simulink model "COGAG"  (Simulink 8.3)
settings: Solver=ode45  StartTime=0.0  StopTime=100.0  FixedStep=0.1  RelTol=1e-3
libraries: simulink_need_slupdate x2
(part 1 of 3)
settings Model: Creator=Administrator  LastModifiedBy=Administrator
settings DataIOCC: SignalLoggingSaveFormat=Dataset  InspectSignalLogs=on
settings DebuggingCC: UnderspecifiedInitializationDetection=Simplified  StateNameClashWarn=none
settings GRTTargetCC: CombineOutputUpdateFcns=on  GRTInterface=off

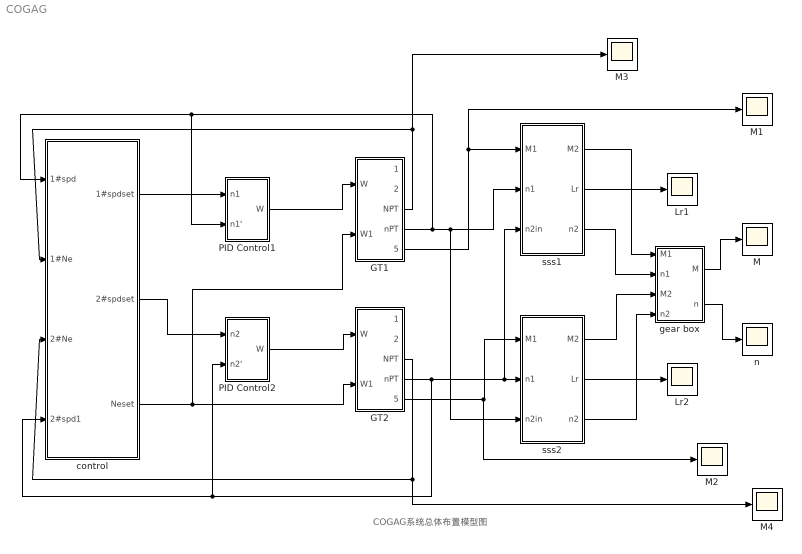
== system COGAG ==
  note: COGAG系统总体布置模型图
  GT1 : Subsystem
  GT2 : Subsystem
  Lr1 : Scope
      settings: YMin=0  YMax=15  SaveName=ScopeData2
  Lr2 : Scope
      settings: SaveName=ScopeData5
  M{,1..4} (5 alike) : Scope
      M settings: SaveName=ScopeData6
      M1 settings: SaveName=ScopeData11
      M2 settings: SaveName=ScopeData12
      M3 settings: SaveName=ScopeData13
      M4 settings: SaveName=ScopeData19
  PID Control1 : Subsystem
  PID Control2 : Subsystem
  control : Subsystem
  gear box : Subsystem
  n : Scope
      settings: SaveName=ScopeData8
  sss1 : Subsystem
  sss2 : Subsystem
  wires:
  GT1/4(nPT) -> sss1/2(n1), sss2/3(n2in), PID Control1/2(n1'), control/1(1#spd)
  GT2/4(nPT) -> control/4(2#spd1), PID Control2/2(n2'), sss2/2(n1), sss1/3(n2in)
  PID Control1/1(W) -> GT1/1(W)
  PID Control2/1(W) -> GT2/1(W)
  control/1(1#spdset) -> PID Control1/1(n1)
  control/2(2#spdset) -> PID Control2/1(n2)
  control/3(Neset) -> GT2/2(W1), GT1/2(W1)
  GT1/3(NPT) -> M3/1, control/2(1#Ne)
  GT2/3(NPT) -> M4/1, control/3(2#Ne)
  GT1/5(MPT) -> M1/1, sss1/1(M1)
  GT2/5(MPT) -> M2/1, sss2/1(M1)
  sss1/2(Lr) -> Lr1/1
  sss2/2(Lr) -> Lr2/1
  gear box/1(M) -> M/1
  gear box/2(n) -> n/1
  sss2/3(n2) -> gear box/4(n2)
  sss1/1(M2) -> gear box/1(M1)
  sss1/3(n2) -> gear box/2(n1)
  sss2/1(M2) -> gear box/3(M2)

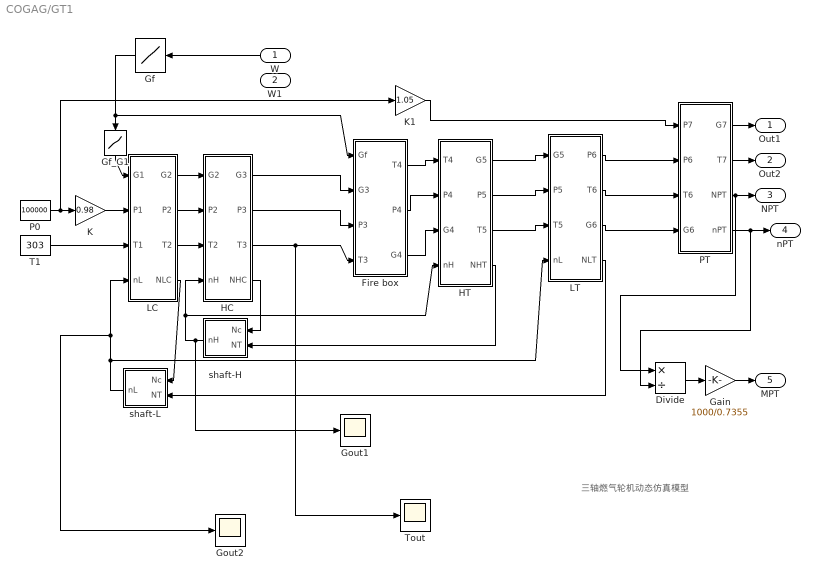
== system COGAG/GT1 ==
  note: 三轴燃气轮机动态仿真模型
  W : Inport
  W1 : Inport  Port=2
  Divide : Product  Inputs=*/
  Fire box : Subsystem
  Gain : Gain  Gain=1000/0.7355
  Gf : Lookup  InputValues=[0,0.03,0.07,0.09,0.11,0.13,0.17,0.2,0.23,0.26,0.28,0.3,0.32,0.34,0.35,0.38,0.4,0.42,0.44,0.47,0.49,0.5,0.52,0.54,0.55,0.59,0.61,0.64,0.66,0.68,0.7,0.72,0.74,0.77,0.81,0.83,0.85,0.88,0.93,0.95,0.97,1]  Table=[0.172,0.236,0.331,0.331,0.366,0.411,0.488,0.536,0.582,0.605,0.644,0.682,0.698,0.728,0.727,0.783,0.783,0.813,0.857,0.886,0.935,0.949,0.95,0.975,0.999,1.022,1.069,1.149,1.153,1.184,1.206,1.233,1.256,1.271,1.325,1.383,1.383,1.439,1.481,1.504,1.52,1.574]
  Gf_G1 : Lookup  InputValues=[0.172,0.236,0.331,0.366,0.411,0.488,0.536,0.582,0.605,0.644,0.682,0.698,0.727,0.728,0.783,0.813,0.857,0.886,0.935,0.949,0.95,0.975,0.999,1.022,1.069,1.149,1.153,1.184,1.206,1.233,1.256,1.271,1.325,1.383,1.439,1.481,1.504,1.52,1.574]  Table="[20.01, 25.93, 38.77,  43.65, 45.94, 51.85, 54.70, 56.85, 59.03, 61.91, 60.44, 61.58, 62.93, 63.04, 65.71,   67.00, 69.52, 70.63, 73.19, 73.46, 73.44, 73.83, 75.62, 76.39, 78.27, 81.17, 81.50, 82.44, 83.44, 84.31, 85.30, 86.17, 87.93, 89.72, 91.51, 93.65, 94.63, 94.92, 97.64]"
  Gout1 : Scope
      settings: TimeRange=10
  Gout2 : Scope
      settings: TimeRange=10  SaveName=ScopeData3
  HC : Subsystem
  HT : Subsystem
  K : Gain  Gain=0.98
  K1 : Gain  Gain=1.05
  LC : Subsystem
  LT : Subsystem
  P0 : Constant  Value=100000
  PT : Subsystem
  T1 : Constant  Value=303
  Tout : Scope
      settings: TimeRange=200  YMin=740  YMax=790
  shaft-H : Subsystem  mask(rotor module){J=30}
      mask prompts: J "J moment of inertia(Nm)"
      mask help: (pi^2*J*n/900)*(dn/dt)=NT-Nc
  shaft-L : Subsystem  mask(rotor module){J=15}
      mask prompts: J "J moment of inertia(Nm)"
      mask help: (pi^2*J*n/900)*(dn/dt)=NT-Nc
  Out1 : Outport
  Out2 : Outport  Port=2
  NPT : Outport  Port=3
  nPT : Outport  Port=4
  MPT : Outport  Port=5
  wires:
  T1/1 -> LC/3(T1)
  K/1 -> LC/2(P1)
  LC/1(G2) -> HC/1(G2)
  LC/2(P2) -> HC/2(P2)
  LC/3(T2) -> HC/3(T2)
  HC/1(G3) -> Fire box/2(G3)
  HC/2(P3) -> Fire box/3(P3)
  HC/3(T3) -> Fire box/4(T3), Tout/1
  HC/4(NHC) -> shaft-H/1(Nc)
  HT/4(NHT) -> shaft-H/2(NT)
  shaft-H/1(nH) -> HT/4(nH), HC/4(nH), Gout1/1
  LC/4(NLC) -> shaft-L/1(Nc)
  LT/4(NLT) -> shaft-L/2(NT)
  Gf/1 -> Gf_G1/1, Fire box/1(Gf)
  Gf_G1/1 -> LC/1(G1)
  Fire box/3(G4) -> HT/3(G4)
  Fire box/2(P4) -> HT/2(P4)
  HT/3(T5) -> LT/3(T5)
  HT/2(P5) -> LT/2(P5)
  HT/1(G5) -> LT/1(G5)
  LT/3(G6) -> PT/4(G6)
  LT/2(T6) -> PT/3(T6)
  shaft-L/1(nL) -> LT/4(nL), LC/4(nL), Gout2/1
  LT/1(P6) -> PT/2(P6)
  P0/1 -> K/1, K1/1
  Fire box/1(T4) -> HT/1(T4)
  K1/1 -> PT/1(P7)
  W/1 -> Gf/1
  PT/1(G7) -> Out1/1
  PT/2(T7) -> Out2/1
  PT/3(NPT) -> NPT/1, Divide/1
  PT/4(nPT) -> nPT/1, Divide/2
  Gain/1 -> MPT/1
  Divide/1 -> Gain/1

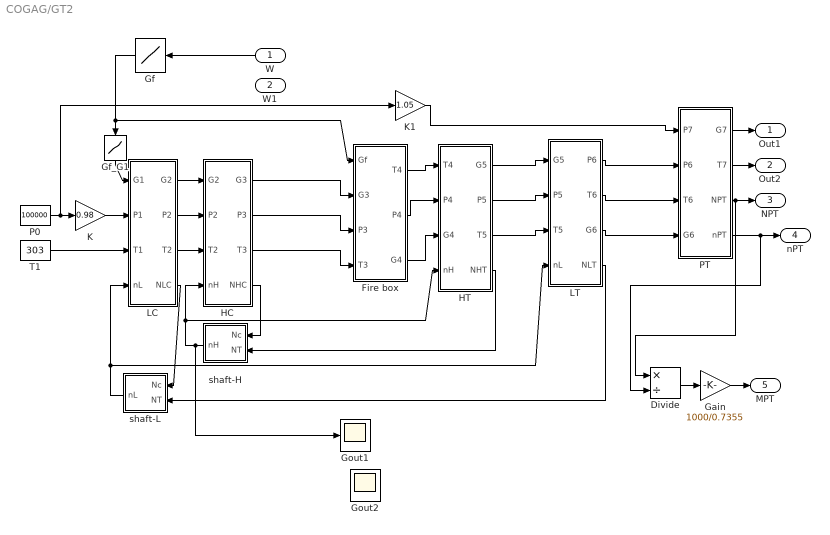
== system COGAG/GT2 ==
  W : Inport
  W1 : Inport  Port=2
  Divide : Product  Inputs=*/
  Fire box : Subsystem
  Gain : Gain  Gain=1000/0.7355
  Gf : Lookup  InputValues=[0,0.03,0.07,0.09,0.11,0.13,0.17,0.2,0.23,0.26,0.28,0.3,0.32,0.34,0.35,0.38,0.4,0.42,0.44,0.47,0.49,0.5,0.52,0.54,0.55,0.59,0.61,0.64,0.66,0.68,0.7,0.72,0.74,0.77,0.81,0.83,0.85,0.88,0.93,0.95,0.97,1]  Table=[0.172,0.236,0.331,0.331,0.366,0.411,0.488,0.536,0.582,0.605,0.644,0.682,0.698,0.728,0.727,0.783,0.783,0.813,0.857,0.886,0.935,0.949,0.95,0.975,0.999,1.022,1.069,1.149,1.153,1.184,1.206,1.233,1.256,1.271,1.325,1.383,1.383,1.439,1.481,1.504,1.52,1.574]
  Gf_G1 : Lookup  InputValues=[0.172,0.236,0.331,0.366,0.411,0.488,0.536,0.582,0.605,0.644,0.682,0.698,0.727,0.728,0.783,0.813,0.857,0.886,0.935,0.949,0.95,0.975,0.999,1.022,1.069,1.149,1.153,1.184,1.206,1.233,1.256,1.271,1.325,1.383,1.439,1.481,1.504,1.52,1.574]  Table="[20.01, 25.93, 38.77,  43.65, 45.94, 51.85, 54.70, 56.85, 59.03, 61.91, 60.44, 61.58, 62.93, 63.04, 65.71,   67.00, 69.52, 70.63, 73.19, 73.46, 73.44, 73.83, 75.62, 76.39, 78.27, 81.17, 81.50, 82.44, 83.44, 84.31, 85.30, 86.17, 87.93, 89.72, 91.51, 93.65, 94.63, 94.92, 97.64]"
  Gout1 : Scope
      settings: TimeRange=10
  Gout2 : Scope
      settings: TimeRange=10  SaveName=ScopeData26
  HC : Subsystem
  HT : Subsystem
  K : Gain  Gain=0.98
  K1 : Gain  Gain=1.05
  LC : Subsystem
  LT : Subsystem
  P0 : Constant  Value=100000
  PT : Subsystem
  T1 : Constant  Value=303
  shaft-H : Subsystem  mask(rotor module){J=30}
      mask prompts: J "J moment of inertia(Nm)"
      mask help: (pi^2*J*n/900)*(dn/dt)=NT-Nc
  shaft-L : Subsystem  mask(rotor module){J=15}
      mask prompts: J "J moment of inertia(Nm)"
      mask help: (pi^2*J*n/900)*(dn/dt)=NT-Nc
  Out1 : Outport
  Out2 : Outport  Port=2
  NPT : Outport  Port=3
  nPT : Outport  Port=4
  MPT : Outport  Port=5
  wires:
  T1/1 -> LC/3(T1)
  K/1 -> LC/2(P1)
  LC/1(G2) -> HC/1(G2)
  LC/2(P2) -> HC/2(P2)
  LC/3(T2) -> HC/3(T2)
  HC/1(G3) -> Fire box/2(G3)
  HC/2(P3) -> Fire box/3(P3)
  HC/3(T3) -> Fire box/4(T3)
  HC/4(NHC) -> shaft-H/1(Nc)
  HT/4(NHT) -> shaft-H/2(NT)
  shaft-H/1(nH) -> HT/4(nH), HC/4(nH), Gout1/1
  LC/4(NLC) -> shaft-L/1(Nc)
  LT/4(NLT) -> shaft-L/2(NT)
  Gf/1 -> Gf_G1/1, Fire box/1(Gf)
  Gf_G1/1 -> LC/1(G1)
  Fire box/3(G4) -> HT/3(G4)
  Fire box/2(P4) -> HT/2(P4)
  HT/3(T5) -> LT/3(T5)
  HT/2(P5) -> LT/2(P5)
  HT/1(G5) -> LT/1(G5)
  LT/3(G6) -> PT/4(G6)
  LT/2(T6) -> PT/3(T6)
  shaft-L/1(nL) -> LT/4(nL), LC/4(nL)
  LT/1(P6) -> PT/2(P6)
  P0/1 -> K/1, K1/1
  Fire box/1(T4) -> HT/1(T4)
  K1/1 -> PT/1(P7)
  W/1 -> Gf/1
  PT/1(G7) -> Out1/1
  PT/2(T7) -> Out2/1
  PT/3(NPT) -> NPT/1, Divide/1
  PT/4(nPT) -> nPT/1, Divide/2
  Gain/1 -> MPT/1
  Divide/1 -> Gain/1

== system COGAG/PID Control1 ==
  note: 模糊自整定PID控制器
  n1 : Inport
  n1' : Inport  Port=2
  Add : Sum  Inputs=+-
  PID Controller : simulink_need_slupdate/PID Controller  P=0.006  I=10  D=0
  Transfer Fcn : TransferFcn  Denominator=[0.6 1]
  W : Outport
  wires:
  Add/1 -> PID Controller/1
  Transfer Fcn/1 -> W/1
  n1/1 -> Add/1
  n1'/1 -> Add/2
  PID Controller/1 -> Transfer Fcn/1

== system COGAG/PID Control2 ==
  n2 : Inport
  n2' : Inport  Port=2
  Add : Sum  Inputs=+-
  PID Controller : simulink_need_slupdate/PID Controller  P=0.006  I=10  D=0
  Transfer Fcn : TransferFcn  Denominator=[0.6 1]
  W : Outport
  wires:
  Add/1 -> PID Controller/1
  PID Controller/1 -> Transfer Fcn/1
  Transfer Fcn/1 -> W/1
  n2/1 -> Add/1
  n2'/1 -> Add/2

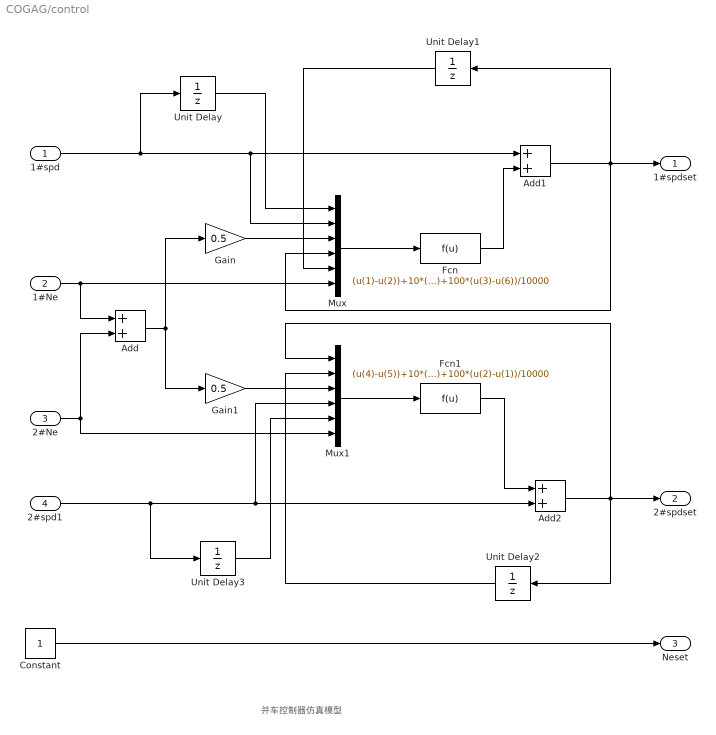
== system COGAG/control ==
  note: 并车控制器仿真模型
  1#spd : Inport
  1#Ne : Inport  Port=2
  2#Ne : Inport  Port=3
  2#spd1 : Inport  Port=4
  Add : Sum
  Add1 : Sum
  Add2 : Sum
  Constant : Constant
  Fcn : Fcn  Expr=(u(1)-u(2))+10*((u(1)-u(2))+u(4)-u(5))+100*(u(3)-u(6))/10000
  Fcn1 : Fcn  Expr=(u(4)-u(5))+10*((u(4)-u(5))+u(4)-u(5))+100*(u(2)-u(1))/10000
  Gain : Gain  Gain=0.5
  Gain1 : Gain  Gain=0.5
  Mux : Mux  Inputs=6
  Mux1 : Mux  Inputs=6
  Unit Delay{,1..3} (4 alike) : UnitDelay  SampleTime=0.02
  1#spdset : Outport
  2#spdset : Outport  Port=2
  Neset : Outport  Port=3
  wires:
  1#Ne/1 -> Add/1, Mux/6
  2#Ne/1 -> Add/2, Mux1/6
  Add/1 -> Gain/1, Gain1/1
  Gain/1 -> Mux/3
  Fcn/1 -> Add1/2
  1#spd/1 -> Unit Delay/1, Add1/1, Mux/2
  Unit Delay/1 -> Mux/1
  Add1/1 -> Mux/4, Unit Delay1/1, 1#spdset/1
  Gain1/1 -> Mux1/3
  Add2/1 -> Unit Delay2/1, 2#spdset/1, Mux1/1
  2#spd1/1 -> Unit Delay3/1, Add2/2, Mux1/4
  Fcn1/1 -> Add2/1
  Unit Delay2/1 -> Mux1/2
  Unit Delay3/1 -> Mux1/5
  Constant/1 -> Neset/1
  Unit Delay1/1 -> Mux/5
  Mux/1 -> Fcn/1
  Mux1/1 -> Fcn1/1

== system COGAG/gear box ==
  note: 并车齿轮箱模型
  M1 : Inport
  n1 : Inport  Port=2
  M2 : Inport  Port=3
  n2 : Inport  Port=4
  Add : Sum
  Fcn : Fcn  Expr=1/u
  Gain : Gain  Gain=1/3.5
  Product : Product
  Product1 : Product
  Product2 : Product
  M : Outport
  n : Outport  Port=2
  wires:
  M1/1 -> Product/1
  n1/1 -> Gain/1, Product/2
  Product/1 -> Add/1
  M2/1 -> Product1/1
  n2/1 -> Product1/2
  Product1/1 -> Add/2
  Gain/1 -> n/1, Fcn/1
  Add/1 -> Product2/1
  Fcn/1 -> Product2/2
  Product2/1 -> M/1

== system COGAG/sss1 ==
  note: sss离合器模块
  M1 : Inport
  n1 : Inport  Port=2
  n2in : Inport  Port=3
  Add : Sum  Inputs=+-
  Fcn : Fcn  Expr=u*pi/30
  Subsystem : Subsystem
  Subsystem1 : Subsystem
  Subsystem2 : Subsystem
  Subsystem3 : Subsystem
  Switch : Switch
  M2 : Outport
  Lr : Outport  Port=2
  n2 : Outport  Port=3
  wires:
  n1/1 -> Subsystem3/2(n1), Switch/1
  Fcn/1 -> Add/2
  Switch/1 -> n2/1
  M1/1 -> Subsystem3/1(M1)
  Subsystem/1(J1) -> Subsystem3/3(J1)
  Subsystem/2(Jz) -> Subsystem1/2(Jz)
  Subsystem3/1(Mfzf) -> Subsystem1/1(Mfzf)
  Subsystem3/3(C1) -> Subsystem1/3(C1)
  Subsystem1/1(Mr) -> Subsystem2/1(Mr)
  Subsystem1/3(C2) -> Subsystem2/3(C2)
  Subsystem1/2(Lr) -> Switch/2, Lr/1
  Subsystem3/2(wf) -> Add/1
  Subsystem/3(J2) -> Subsystem2/2(J2)
  Subsystem2/1(M2) -> M2/1
  Subsystem/4(f) -> Subsystem1/4(f)
  n2in/1 -> Subsystem2/4(n2in)
  Add/1 -> Subsystem1/5(Wz)
  Subsystem2/2(n2) -> Fcn/1, Switch/3

== system COGAG/sss2 ==
  note: sss离合器模块
  M1 : Inport
  n1 : Inport  Port=2
  n2in : Inport  Port=3
  Add : Sum  Inputs=+-
  Fcn : Fcn  Expr=u*pi/30
  Subsystem : Subsystem
  Subsystem1 : Subsystem
  Subsystem2 : Subsystem
  Subsystem3 : Subsystem
  Switch : Switch
  M2 : Outport
  Lr : Outport  Port=2
  n2 : Outport  Port=3
  wires:
  n1/1 -> Subsystem3/2(n1), Switch/1
  Fcn/1 -> Add/2
  Switch/1 -> n2/1
  M1/1 -> Subsystem3/1(M1)
  Subsystem/1(J1) -> Subsystem3/3(J1)
  Subsystem/2(Jz) -> Subsystem1/2(Jz)
  Subsystem3/1(Mfzf) -> Subsystem1/1(Mfzf)
  Subsystem3/3(C1) -> Subsystem1/3(C1)
  Subsystem1/1(Mr) -> Subsystem2/1(Mr)
  Subsystem1/3(C2) -> Subsystem2/3(C2)
  Subsystem1/2(Lr) -> Switch/2, Lr/1
  Subsystem3/2(wf) -> Add/1
  Subsystem/3(J2) -> Subsystem2/2(J2)
  Subsystem2/1(M2) -> M2/1
  Subsystem/4(f) -> Subsystem1/4(f)
  n2in/1 -> Subsystem2/4(n2in)
  Add/1 -> Subsystem1/5(Wz)
  Subsystem2/2(n2) -> Fcn/1, Switch/3

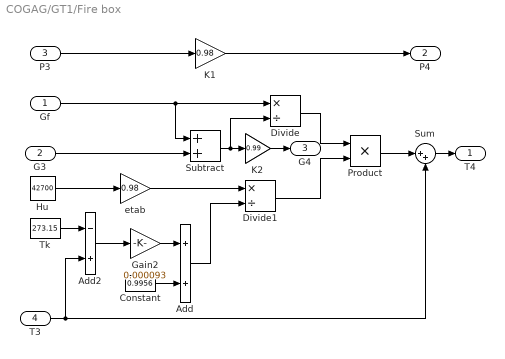
== system COGAG/GT1/Fire box ==
  Gf : Inport
  G3 : Inport  Port=2
  P3 : Inport  Port=3
  T3 : Inport  Port=4
  Add : Sum
  Add2 : Sum  Inputs=-+
  Constant : Constant  Value=0.9956
  Divide : Product  Inputs=*/
  Divide1 : Product  Inputs=*/
  Gain2 : Gain  Gain=0.000093
  Hu : Constant  Value=42700
  K1 : Gain  Gain=0.98
  K2 : Gain  Gain=0.99
  Product : Product  RndMeth=Zero
  Subtract : Sum
  Sum : Sum  Inputs=|++
  Tk : Constant  Value=273.15
  etab : Gain  Gain=0.98
  T4 : Outport
  P4 : Outport  Port=2
  G4 : Outport  Port=3
  wires:
  Gf/1 -> Divide/1, Subtract/1
  Divide/1 -> Product/1
  G3/1 -> Subtract/2
  Subtract/1 -> Divide/2, K2/1
  Hu/1 -> etab/1
  etab/1 -> Divide1/1
  Divide1/1 -> Product/2
  Product/1 -> Sum/1
  Sum/1 -> T4/1
  T3/1 -> Add2/2, Sum/2
  P3/1 -> K1/1
  K1/1 -> P4/1
  Constant/1 -> Add/2
  Gain2/1 -> Add/1
  Tk/1 -> Add2/1
  Add2/1 -> Gain2/1
  Add/1 -> Divide1/2
  K2/1 -> G4/1

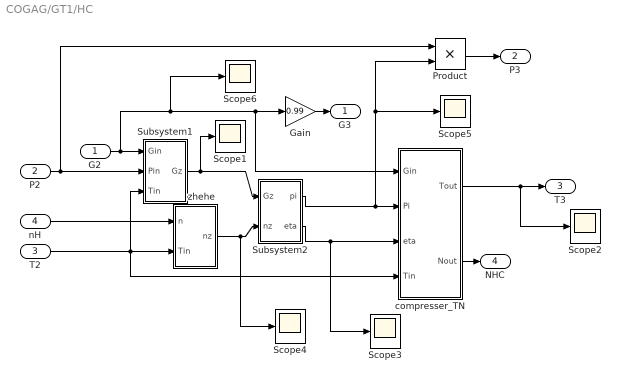
== system COGAG/GT1/HC ==
  G2 : Inport
  P2 : Inport  Port=2
  T2 : Inport  Port=3
  nH : Inport  Port=4
  Gain : Gain  Gain=0.99
  Product : Product  RndMeth=Zero
  Scope{1..6} (6 alike) : Scope
      Scope1 settings: YMin=2829.54  YMax=3127.38  SaveName=ScopeData16
      Scope2 settings: YMin=2829.54  YMax=3127.38  SaveName=ScopeData29
      Scope3 settings: YMin=2829.54  YMax=3127.38  SaveName=ScopeData24
      Scope4 settings: YMin=2829.54  YMax=3127.38  SaveName=ScopeData31
      Scope5 settings: YMin=2829.54  YMax=3127.38  SaveName=ScopeData10
      Scope6 settings: YMin=2829.54  YMax=3127.38  SaveName=ScopeData15
  Subsystem1 : Subsystem
  Subsystem2 : Subsystem
  compresser_TN : Subsystem  mask(Compressor_Tout Nout module){}
  zhehe : Subsystem
  G3 : Outport
  P3 : Outport  Port=2
  T3 : Outport  Port=3
  NHC : Outport  Port=4
  wires:
  zhehe/1(nz) -> Scope4/1, Subsystem2/2(nz)
  Subsystem2/1(pi) -> compresser_TN/2(Pi), Product/2, Scope5/1
  Subsystem2/2(eta) -> compresser_TN/3(eta), Scope3/1
  T2/1 -> zhehe/2(Tin), compresser_TN/4(Tin), Subsystem1/3(Tin)
  nH/1 -> zhehe/1(n)
  Gain/1 -> G3/1
  compresser_TN/1(Tout) -> T3/1, Scope2/1
  compresser_TN/2(Nout) -> NHC/1
  Subsystem1/1(Gz) -> Scope1/1, Subsystem2/1(Gz)
  G2/1 -> Subsystem1/1(Gin), Gain/1, compresser_TN/1(Gin), Scope6/1
  P2/1 -> Subsystem1/2(Pin), Product/1
  Product/1 -> P3/1

== system COGAG/GT1/HT ==
  T4 : Inport
  P4 : Inport  Port=2
  G4 : Inport  Port=3
  nH : Inport  Port=4
  Divide : Product  Inputs=*/
  Scope3 : Scope
      settings: TimeRange=100  YMin=5000  YMax=25000  SaveName=ScopeData34
  n2-etaH : Lookup  InputValues=[6000 6300 6500 6800 7000 7150 7300 7500 7800]  Table=[0.81 0.83 0.85 0.87 0.88 0.87 0.86 0.855 0.85]
  n2-p1 : Lookup  InputValues=[6000 6503 6995 7498 8002 8505 8997 9500]  Table=[139400 150700 186000 246700 332500 443400 575800 736100]
  n2-p5 : Lookup  InputValues=[5832,7212,7282,7644,7752,7853,8033,8092 8211 8392 8430 8452 8670 8767 8960 8999 9073]  Table=[154000,269000,296000,361000,391000,419000,476000,494000 534000 596000 609000 616000 684000 719000 806000 814000 831000]
  pi : Scope
      settings: TimeRange=100  YMin=2829.54  YMax=3127.38  SaveName=ScopeData17
  pi1 : Scope
      settings: TimeRange=100  YMin=2829.54  YMax=3127.38  SaveName=ScopeData7
  pi2 : Scope
      settings: TimeRange=100  YMin=2829.54  YMax=3127.38  SaveName=ScopeData35
  turbine_TN : Subsystem  mask(Turbine_Tout Nout module){}
  G5 : Outport
  P5 : Outport  Port=2
  T5 : Outport  Port=3
  NHT : Outport  Port=4
  wires:
  n2-etaH/1 -> turbine_TN/2(eta)
  P4/1 -> Divide/1
  nH/1 -> pi2/1, n2-etaH/1, n2-p5/1
  turbine_TN/1(Tout) -> T5/1, pi1/1
  T4/1 -> turbine_TN/3(Tin)
  turbine_TN/2(Nout) -> NHT/1
  G4/1 -> turbine_TN/4(Gin), G5/1
  Divide/1 -> turbine_TN/1(Pi), pi/1
  n2-p5/1 -> Divide/2, P5/1, Scope3/1

== system COGAG/GT1/LC ==
  G1 : Inport
  P1 : Inport  Port=2
  T1 : Inport  Port=3
  nL : Inport  Port=4
  Gain : Gain  Gain=0.99
  Product : Product  RndMeth=Zero
  Scope{1..4} (4 alike) : Scope
      Scope1 settings: YMin=2829.54  YMax=3127.38  SaveName=ScopeData14
      Scope2 settings: YMin=2829.54  YMax=3127.38  SaveName=ScopeData9
      Scope3 settings: YMin=2829.54  YMax=3127.38  SaveName=ScopeData30
      Scope4 settings: TimeRange=80  YMin=5000  YMax=30000  SaveName=ScopeData32
  Subsystem1 : Subsystem
  Subsystem3 : Subsystem
  compresser_TN : Subsystem  mask(Compressor_Tout Nout module){}
  zhehe : Subsystem
  G2 : Outport
  P2 : Outport  Port=2
  T2 : Outport  Port=3
  NLC : Outport  Port=4
  wires:
  zhehe/1(nz) -> Scope1/1, Subsystem3/2(nz)
  Subsystem3/1(pi) -> compresser_TN/2(Pi), Product/2, Scope2/1
  Subsystem3/2(eta) -> compresser_TN/3(eta)
  T1/1 -> zhehe/2(Tin), compresser_TN/4(Tin), Subsystem1/3(Tin)
  nL/1 -> zhehe/1(n)
  Gain/1 -> G2/1
  compresser_TN/1(Tout) -> T2/1, Scope4/1
  compresser_TN/2(Nout) -> NLC/1
  Subsystem1/1(Gz) -> Scope3/1, Subsystem3/1(Gz)
  G1/1 -> Subsystem1/1(Gin), Gain/1, compresser_TN/1(Gin)
  P1/1 -> Subsystem1/2(Pin), Product/1
  Product/1 -> P2/1

== system COGAG/GT1/LT ==
  G5 : Inport
  P5 : Inport  Port=2
  T5 : Inport  Port=3
  nL : Inport  Port=4
  Divide : Product  Inputs=*/
  Scope1 : Scope
      settings: TimeRange=100  YMin=5000  YMax=25000  SaveName=ScopeData28
  Scope2 : Scope
      settings: TimeRange=100  YMin=5000  YMax=25000  SaveName=ScopeData4
  Scope3 : Scope
      settings: TimeRange=100  YMin=5000  YMax=25000  SaveName=ScopeData20
  n1-p1 : Lookup  InputValues="[2849,4651,4850,5410,5586,5742,6024,6092,6102,6211,6385,6425 6435 6609 6698  6732 7015  7080 7185 ]"  Table="[101000,131000,141000,161000,171000,181000,201000,201000,211000,221000,241000,251000 251000 281000 291000  301000 321000  331000 341000]"
  n1-p6 : Lookup  InputValues=[2849,4651,4850,5410,5586,5742,6024,6092,6102,6211,6385,6425,6435,6609,6698,6732,7015,7080,7185]  Table=[113000,150000,157000,180000,190000,201000,221000,229000,229500,242000,267000,272000,277000,306000,321000,322000,354000,360000,371000]
  n2-etaH : Lookup  InputValues=[4300 5000 5500 6000 6500 7000 7500 8000 9000 9500]  Table=[0.82 0.83 0.835 0.84 0.85 0.86 0.875 0.87 0.865 0.86]
  turbine_TN : Subsystem  mask(Turbine_Tout Nout module){}
  P6 : Outport
  T6 : Outport  Port=2
  G6 : Outport  Port=3
  NLT : Outport  Port=4
  wires:
  n2-etaH/1 -> turbine_TN/2(eta)
  P5/1 -> Divide/1
  nL/1 -> n2-etaH/1, n1-p6/1
  turbine_TN/1(Tout) -> T6/1, Scope2/1
  T5/1 -> turbine_TN/3(Tin)
  turbine_TN/2(Nout) -> NLT/1
  G5/1 -> turbine_TN/4(Gin), G6/1
  n1-p6/1 -> Divide/2, P6/1, Scope1/1
  Divide/1 -> turbine_TN/1(Pi), Scope3/1

== system COGAG/GT1/PT ==
  P7 : Inport
  P6 : Inport  Port=2
  T6 : Inport  Port=3
  G6 : Inport  Port=4
  Divide : Product  Inputs=*/
  Pi-eta1 : Lookup  InputValues=[1,1.11 1.41 1.51 1.81 2.0 2.21 2.41 2.61 2.81]  Table=[0.825,0.83 0.85 0.86 0.88 0.90 0.905 0.91 0.905 0.9]
  Pi-eta2 : Lookup  InputValues=[307,625,1634,2141,2611,3121,4030,4941,5687,6256,6755,7309,7716,8175,8374,9153,9719,10196,10702,11284,11832,12033,12512,13051,13298,14334,14778,15580,16003,16531,16669,17381,17948,18600,19648,20212,20613,21462,22525,23139,23520,24372]  Table=[878,1243,1778,1749,1547,1574,1765,1930,2049,2045,2069,2150,2158,2185,2214,2272,2274,2209,2231,2240,2252,2500,2569,2649,2574,2650,2617,2639,2697,2653,2702,2785,2901,2979,3042,2919,2951,3108,3089,3056,3065,3142]
  Scope6 : Scope
      settings: YMin=2829.54  YMax=3127.38  SaveName=ScopeData22
  turbine_TN : Subsystem  mask(Turbine_Tout Nout module){}
  G7 : Outport
  T7 : Outport  Port=2
  NPT : Outport  Port=3
  nPT : Outport  Port=4
  wires:
  turbine_TN/1(Tout) -> T7/1
  turbine_TN/2(Nout) -> NPT/1, Pi-eta2/1
  G6/1 -> turbine_TN/3(Gin), G7/1
  Divide/1 -> Scope6/1, turbine_TN/1(Pi), Pi-eta1/1
  T6/1 -> turbine_TN/4(Tin)
  Pi-eta1/1 -> turbine_TN/2(eta)
  P6/1 -> Divide/1
  P7/1 -> Divide/2
  Pi-eta2/1 -> nPT/1

== system COGAG/GT1/shaft-H ==
  Nc : Inport
  NT : Inport  Port=2
  Add : Sum  Inputs=-+
  Divide : Product  Inputs=3
  Fcn : Fcn  Expr=1/u
  Fcn1 : Fcn  Expr=1/u
  Gain : Gain  Gain=15/(pi*pi)
  Gain3 : Gain  Gain=60
  Integrator : Integrator  InitialCondition=143.58
  J : Constant  Value=J
  nH : Outport
  wires:
  Nc/1 -> Add/1
  NT/1 -> Add/2
  Divide/1 -> Integrator/1
  Integrator/1 -> Fcn1/1, Gain3/1
  Add/1 -> Divide/1
  J/1 -> Fcn/1
  Gain/1 -> Divide/2
  Fcn/1 -> Gain/1
  Fcn1/1 -> Divide/3
  Gain3/1 -> nH/1

== system COGAG/GT1/shaft-L ==
  Nc : Inport
  NT : Inport  Port=2
  Add : Sum  Inputs=-+
  Divide : Product  Inputs=3
  Fcn : Fcn  Expr=1/u
  Fcn1 : Fcn  Expr=1/u
  Gain : Gain  Gain=15/(pi*pi)
  Gain2 : Gain  Gain=60
  Integrator : Integrator  InitialCondition=105.9
  J : Constant  Value=J
  nL : Outport
  wires:
  Nc/1 -> Add/1
  NT/1 -> Add/2
  Divide/1 -> Integrator/1
  Integrator/1 -> Fcn1/1, Gain2/1
  Add/1 -> Divide/1
  J/1 -> Fcn/1
  Gain/1 -> Divide/2
  Fcn/1 -> Gain/1
  Fcn1/1 -> Divide/3
  Gain2/1 -> nL/1

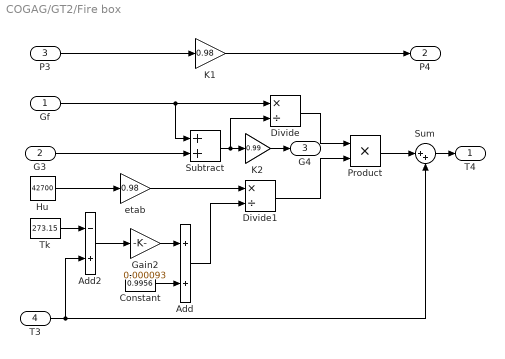
== system COGAG/GT2/Fire box ==
  Gf : Inport
  G3 : Inport  Port=2
  P3 : Inport  Port=3
  T3 : Inport  Port=4
  Add : Sum
  Add2 : Sum  Inputs=-+
  Constant : Constant  Value=0.9956
  Divide : Product  Inputs=*/
  Divide1 : Product  Inputs=*/
  Gain2 : Gain  Gain=0.000093
  Hu : Constant  Value=42700
  K1 : Gain  Gain=0.98
  K2 : Gain  Gain=0.99
  Product : Product  RndMeth=Zero
  Subtract : Sum
  Sum : Sum  Inputs=|++
  Tk : Constant  Value=273.15
  etab : Gain  Gain=0.98
  T4 : Outport
  P4 : Outport  Port=2
  G4 : Outport  Port=3
  wires:
  Gf/1 -> Divide/1, Subtract/1
  Divide/1 -> Product/1
  G3/1 -> Subtract/2
  Subtract/1 -> Divide/2, K2/1
  Hu/1 -> etab/1
  etab/1 -> Divide1/1
  Divide1/1 -> Product/2
  Product/1 -> Sum/1
  Sum/1 -> T4/1
  T3/1 -> Add2/2, Sum/2
  P3/1 -> K1/1
  K1/1 -> P4/1
  Constant/1 -> Add/2
  Gain2/1 -> Add/1
  Tk/1 -> Add2/1
  Add2/1 -> Gain2/1
  Add/1 -> Divide1/2
  K2/1 -> G4/1

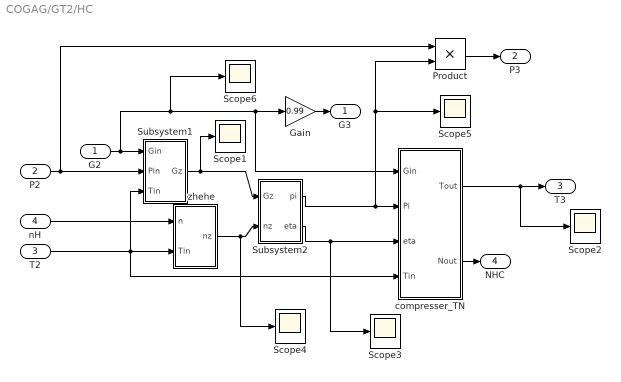
== system COGAG/GT2/HC ==
  G2 : Inport
  P2 : Inport  Port=2
  T2 : Inport  Port=3
  nH : Inport  Port=4
  Gain : Gain  Gain=0.99
  Product : Product  RndMeth=Zero
  Scope{1..6} (6 alike) : Scope
      Scope1 settings: YMin=2829.54  YMax=3127.38  SaveName=ScopeData16
      Scope2 settings: YMin=2829.54  YMax=3127.38  SaveName=ScopeData29
      Scope3 settings: YMin=2829.54  YMax=3127.38  SaveName=ScopeData24
      Scope4 settings: YMin=2829.54  YMax=3127.38  SaveName=ScopeData31
      Scope5 settings: YMin=2829.54  YMax=3127.38  SaveName=ScopeData10
      Scope6 settings: YMin=2829.54  YMax=3127.38  SaveName=ScopeData15
  Subsystem1 : Subsystem
  Subsystem2 : Subsystem
  compresser_TN : Subsystem  mask(Compressor_Tout Nout module){}
  zhehe : Subsystem
  G3 : Outport
  P3 : Outport  Port=2
  T3 : Outport  Port=3
  NHC : Outport  Port=4
  wires:
  zhehe/1(nz) -> Scope4/1, Subsystem2/2(nz)
  Subsystem2/1(pi) -> compresser_TN/2(Pi), Product/2, Scope5/1
  Subsystem2/2(eta) -> compresser_TN/3(eta), Scope3/1
  T2/1 -> zhehe/2(Tin), compresser_TN/4(Tin), Subsystem1/3(Tin)
  nH/1 -> zhehe/1(n)
  Gain/1 -> G3/1
  compresser_TN/1(Tout) -> T3/1, Scope2/1
  compresser_TN/2(Nout) -> NHC/1
  Subsystem1/1(Gz) -> Scope1/1, Subsystem2/1(Gz)
  G2/1 -> Subsystem1/1(Gin), Gain/1, compresser_TN/1(Gin), Scope6/1
  P2/1 -> Subsystem1/2(Pin), Product/1
  Product/1 -> P3/1

== system COGAG/GT2/HT ==
  T4 : Inport
  P4 : Inport  Port=2
  G4 : Inport  Port=3
  nH : Inport  Port=4
  Divide : Product  Inputs=*/
  Scope3 : Scope
      settings: TimeRange=100  YMin=5000  YMax=25000  SaveName=ScopeData34
  n2-etaH : Lookup  InputValues=[6000 6300 6500 6800 7000 7150 7300 7500 7800]  Table=[0.81 0.83 0.85 0.87 0.88 0.87 0.86 0.855 0.85]
  n2-p1 : Lookup  InputValues=[6000 6503 6995 7498 8002 8505 8997 9500]  Table=[139400 150700 186000 246700 332500 443400 575800 736100]
  n2-p5 : Lookup  InputValues=[5832,7212,7282,7644,7752,7853,8033,8092 8211 8392 8430 8452 8670 8767 8960 8999 9073]  Table=[154000,269000,296000,361000,391000,419000,476000,494000 534000 596000 609000 616000 684000 719000 806000 814000 831000]
  pi : Scope
      settings: TimeRange=100  YMin=2829.54  YMax=3127.38  SaveName=ScopeData17
  pi1 : Scope
      settings: TimeRange=100  YMin=2829.54  YMax=3127.38  SaveName=ScopeData7
  pi2 : Scope
      settings: TimeRange=100  YMin=2829.54  YMax=3127.38  SaveName=ScopeData35
  turbine_TN : Subsystem  mask(Turbine_Tout Nout module){}
  G5 : Outport
  P5 : Outport  Port=2
  T5 : Outport  Port=3
  NHT : Outport  Port=4
  wires:
  n2-etaH/1 -> turbine_TN/2(eta)
  P4/1 -> Divide/1
  nH/1 -> pi2/1, n2-etaH/1, n2-p5/1
  turbine_TN/1(Tout) -> T5/1, pi1/1
  T4/1 -> turbine_TN/3(Tin)
  turbine_TN/2(Nout) -> NHT/1
  G4/1 -> turbine_TN/4(Gin), G5/1
  Divide/1 -> turbine_TN/1(Pi), pi/1
  n2-p5/1 -> Divide/2, P5/1, Scope3/1

== system COGAG/GT2/LC ==
  G1 : Inport
  P1 : Inport  Port=2
  T1 : Inport  Port=3
  nL : Inport  Port=4
  Gain : Gain  Gain=0.99
  Product : Product  RndMeth=Zero
  Scope{1..4} (4 alike) : Scope
      Scope1 settings: YMin=2829.54  YMax=3127.38  SaveName=ScopeData14
      Scope2 settings: YMin=2829.54  YMax=3127.38  SaveName=ScopeData9
      Scope3 settings: YMin=2829.54  YMax=3127.38  SaveName=ScopeData30
      Scope4 settings: TimeRange=80  YMin=5000  YMax=30000  SaveName=ScopeData32
  Subsystem1 : Subsystem
  Subsystem3 : Subsystem
  compresser_TN : Subsystem  mask(Compressor_Tout Nout module){}
  zhehe : Subsystem
  G2 : Outport
  P2 : Outport  Port=2
  T2 : Outport  Port=3
  NLC : Outport  Port=4
  wires:
  zhehe/1(nz) -> Scope1/1, Subsystem3/2(nz)
  Subsystem3/1(pi) -> compresser_TN/2(Pi), Product/2, Scope2/1
  Subsystem3/2(eta) -> compresser_TN/3(eta)
  T1/1 -> zhehe/2(Tin), compresser_TN/4(Tin), Subsystem1/3(Tin)
  nL/1 -> zhehe/1(n)
  Gain/1 -> G2/1
  compresser_TN/1(Tout) -> T2/1, Scope4/1
  compresser_TN/2(Nout) -> NLC/1
  Subsystem1/1(Gz) -> Scope3/1, Subsystem3/1(Gz)
  G1/1 -> Subsystem1/1(Gin), Gain/1, compresser_TN/1(Gin)
  P1/1 -> Subsystem1/2(Pin), Product/1
  Product/1 -> P2/1

== system COGAG/GT2/LT ==
  G5 : Inport
  P5 : Inport  Port=2
  T5 : Inport  Port=3
  nL : Inport  Port=4
  Divide : Product  Inputs=*/
  Scope1 : Scope
      settings: TimeRange=100  YMin=5000  YMax=25000  SaveName=ScopeData28
  Scope2 : Scope
      settings: TimeRange=100  YMin=5000  YMax=25000  SaveName=ScopeData4
  Scope3 : Scope
      settings: TimeRange=100  YMin=5000  YMax=25000  SaveName=ScopeData20
  n1-p1 : Lookup  InputValues="[2849,4651,4850,5410,5586,5742,6024,6092,6102,6211,6385,6425 6435 6609 6698  6732 7015  7080 7185 ]"  Table="[101000,131000,141000,161000,171000,181000,201000,201000,211000,221000,241000,251000 251000 281000 291000  301000 321000  331000 341000]"
  n1-p6 : Lookup  InputValues=[2849,4651,4850,5410,5586,5742,6024,6092,6102,6211,6385,6425,6435,6609,6698,6732,7015,7080,7185]  Table=[113000,150000,157000,180000,190000,201000,221000,229000,229500,242000,267000,272000,277000,306000,321000,322000,354000,360000,371000]
  n2-etaH : Lookup  InputValues=[4300 5000 5500 6000 6500 7000 7500 8000 9000 9500]  Table=[0.82 0.83 0.835 0.84 0.85 0.86 0.875 0.87 0.865 0.86]
  turbine_TN : Subsystem  mask(Turbine_Tout Nout module){}
  P6 : Outport
  T6 : Outport  Port=2
  G6 : Outport  Port=3
  NLT : Outport  Port=4
  wires:
  n2-etaH/1 -> turbine_TN/2(eta)
  P5/1 -> Divide/1
  nL/1 -> n2-etaH/1, n1-p6/1
  turbine_TN/1(Tout) -> T6/1, Scope2/1
  T5/1 -> turbine_TN/3(Tin)
  turbine_TN/2(Nout) -> NLT/1
  G5/1 -> turbine_TN/4(Gin), G6/1
  n1-p6/1 -> Divide/2, P6/1, Scope1/1
  Divide/1 -> turbine_TN/1(Pi), Scope3/1

== system COGAG/GT2/PT ==
  P7 : Inport
  P6 : Inport  Port=2
  T6 : Inport  Port=3
  G6 : Inport  Port=4
  Divide : Product  Inputs=*/
  Pi-eta1 : Lookup  InputValues=[1,1.11 1.41 1.51 1.81 2.0 2.21 2.41 2.61 2.81]  Table=[0.825,0.83 0.85 0.86 0.88 0.90 0.905 0.91 0.905 0.9]
  Pi-eta2 : Lookup  InputValues=[307,625,1634,2141,2611,3121,4030,4941,5687,6256,6755,7309,7716,8175,8374,9153,9719,10196,10702,11284,11832,12033,12512,13051,13298,14334,14778,15580,16003,16531,16669,17381,17948,18600,19648,20212,20613,21462,22525,23139,23520,24372]  Table=[878,1243,1778,1749,1547,1574,1765,1930,2049,2045,2069,2150,2158,2185,2214,2272,2274,2209,2231,2240,2252,2500,2569,2649,2574,2650,2617,2639,2697,2653,2702,2785,2901,2979,3042,2919,2951,3108,3089,3056,3065,3142]
  Scope6 : Scope
      settings: YMin=2829.54  YMax=3127.38  SaveName=ScopeData22
  turbine_TN : Subsystem  mask(Turbine_Tout Nout module){}
  G7 : Outport
  T7 : Outport  Port=2
  NPT : Outport  Port=3
  nPT : Outport  Port=4
  wires:
  turbine_TN/1(Tout) -> T7/1
  turbine_TN/2(Nout) -> NPT/1, Pi-eta2/1
  G6/1 -> turbine_TN/3(Gin), G7/1
  Divide/1 -> Scope6/1, turbine_TN/1(Pi), Pi-eta1/1
  T6/1 -> turbine_TN/4(Tin)
  Pi-eta1/1 -> turbine_TN/2(eta)
  P6/1 -> Divide/1
  P7/1 -> Divide/2
  Pi-eta2/1 -> nPT/1

== system COGAG/GT2/shaft-H ==
  Nc : Inport
  NT : Inport  Port=2
  Add : Sum  Inputs=-+
  Divide : Product  Inputs=3
  Fcn : Fcn  Expr=1/u
  Fcn1 : Fcn  Expr=1/u
  Gain : Gain  Gain=15/(pi*pi)
  Gain3 : Gain  Gain=60
  Integrator : Integrator  InitialCondition=143.58
  J : Constant  Value=J
  nH : Outport
  wires:
  Nc/1 -> Add/1
  NT/1 -> Add/2
  Divide/1 -> Integrator/1
  Integrator/1 -> Fcn1/1, Gain3/1
  Add/1 -> Divide/1
  J/1 -> Fcn/1
  Gain/1 -> Divide/2
  Fcn/1 -> Gain/1
  Fcn1/1 -> Divide/3
  Gain3/1 -> nH/1

== system COGAG/GT2/shaft-L ==
  Nc : Inport
  NT : Inport  Port=2
  Add : Sum  Inputs=-+
  Divide : Product  Inputs=3
  Fcn : Fcn  Expr=1/u
  Fcn1 : Fcn  Expr=1/u
  Gain : Gain  Gain=15/(pi*pi)
  Gain2 : Gain  Gain=60
  Integrator : Integrator  InitialCondition=105.9
  J : Constant  Value=J
  nL : Outport
  wires:
  Nc/1 -> Add/1
  NT/1 -> Add/2
  Divide/1 -> Integrator/1
  Integrator/1 -> Fcn1/1, Gain2/1
  Add/1 -> Divide/1
  J/1 -> Fcn/1
  Gain/1 -> Divide/2
  Fcn/1 -> Gain/1
  Fcn1/1 -> Divide/3
  Gain2/1 -> nL/1

== system COGAG/sss1/Subsystem ==
  note: 阻尼系数模块
  J : Constant  Value=0.119507
  J2l : Constant  Value=0.092495
  Jk : Constant  Value=0.0694875
  f1 : Constant  Value=0.6
  J1 : Outport
  Jz : Outport  Port=2
  J2 : Outport  Port=3
  f : Outport  Port=4
  wires:
  J/1 -> J1/1
  Jk/1 -> Jz/1
  J2l/1 -> J2/1
  f1/1 -> f/1

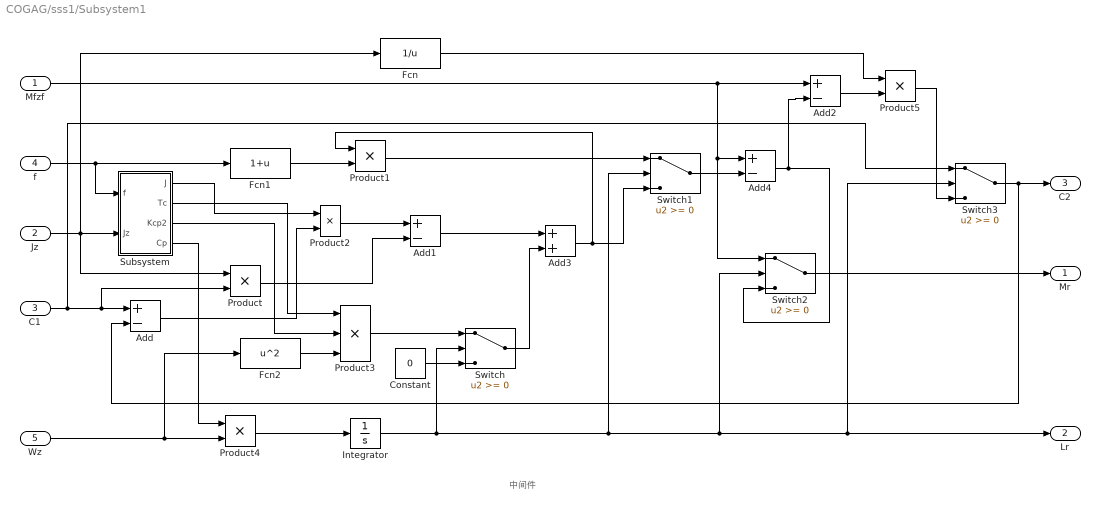
== system COGAG/sss1/Subsystem1 ==
  note: 中间件
  Mfzf : Inport
  Jz : Inport  Port=2
  C1 : Inport  Port=3
  f : Inport  Port=4
  Wz : Inport  Port=5
  Add{,1..2,4} (4 alike) : Sum  Inputs=+-
  Add3 : Sum
  Constant : Constant  Value=0
  Fcn : Fcn  Expr=1/u
  Fcn1 : Fcn  Expr=1+u
  Fcn2 : Fcn  Expr=u^2
  Integrator : Integrator
  Product{,1..2,4..5} (5 alike) : Product
  Product3 : Product  Inputs=3
  Subsystem : Subsystem
  Switch{,1..3} (4 alike) : Switch
  Mr : Outport
  Lr : Outport  Port=2
  C2 : Outport  Port=3
  wires:
  C1/1 -> Switch3/1, Product/2, Add/1
  f/1 -> Subsystem/1(f), Fcn1/1
  Fcn1/1 -> Product1/2
  Product1/1 -> Switch1/1
  Switch1/1 -> Add4/2
  Mfzf/1 -> Add2/1, Add4/1, Switch2/1
  Add2/1 -> Product5/2
  Fcn/1 -> Product5/1
  Switch2/1 -> Mr/1
  Add4/1 -> Add2/2, Switch2/3
  Jz/1 -> Product/1, Subsystem/2(Jz), Fcn/1
  Wz/1 -> Fcn2/1, Product4/2
  Fcn2/1 -> Product3/3
  Integrator/1 -> Lr/1, Switch3/2, Switch2/2, Switch1/2, Switch/2
  Product3/1 -> Switch/1
  Constant/1 -> Switch/3
  Add1/1 -> Add3/1
  Switch/1 -> Add3/2
  Add3/1 -> Product1/1, Switch1/3
  Product/1 -> Add1/2
  Product2/1 -> Add1/1
  Add/1 -> Product2/2
  Subsystem/4(Cp) -> Product4/1
  Subsystem/3(Kcp2) -> Product3/2
  Subsystem/1(J) -> Product2/1
  Subsystem/2(Tc) -> Product3/1
  Product4/1 -> Integrator/1
  Switch3/1 -> Add/2, C2/1
  Product5/1 -> Switch3/3

== system COGAG/sss1/Subsystem2 ==
  note: 从动件
  Mr : Inport
  J2 : Inport  Port=2
  C2 : Inport  Port=3
  n2in : Inport  Port=4
  Add : Sum  Inputs=+-
  Add1 : Sum
  Fcn : Fcn  Expr=30*u/pi
  Integrator : Integrator
  Product : Product
  M2 : Outport
  n2 : Outport  Port=2
  wires:
  Mr/1 -> Add/1
  Add/1 -> M2/1
  J2/1 -> Product/1
  Integrator/1 -> Add1/1
  n2in/1 -> Add1/2
  Add1/1 -> n2/1
  Product/1 -> Add/2
  Fcn/1 -> Integrator/1
  C2/1 -> Fcn/1, Product/2

== system COGAG/sss1/Subsystem3 ==
  note: 主动件
  M1 : Inport
  n1 : Inport  Port=2
  J1 : Inport  Port=3
  Derivative : Derivative
  Fcn2 : Fcn  Expr=u*pi/30
  Product : Product
  Sum : Sum  Inputs=|+-
  Mfzf : Outport
  wf : Outport  Port=2
  C1 : Outport  Port=3
  wires:
  n1/1 -> Fcn2/1
  Fcn2/1 -> wf/1, Derivative/1
  M1/1 -> Sum/1
  J1/1 -> Product/2
  Derivative/1 -> Product/1, C1/1
  Product/1 -> Sum/2
  Sum/1 -> Mfzf/1

== system COGAG/sss2/Subsystem ==
  J : Constant  Value=0.119507
  J2l : Constant  Value=0.092495
  Jk : Constant  Value=0.0694875
  f1 : Constant  Value=0.6
  J1 : Outport
  Jz : Outport  Port=2
  J2 : Outport  Port=3
  f : Outport  Port=4
  wires:
  J/1 -> J1/1
  Jk/1 -> Jz/1
  J2l/1 -> J2/1
  f1/1 -> f/1

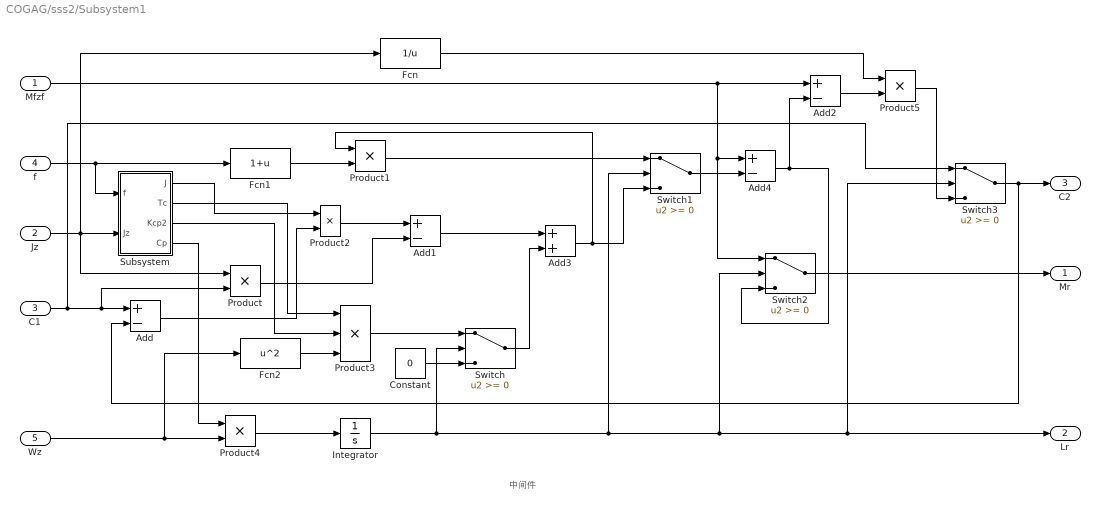
== system COGAG/sss2/Subsystem1 ==
  note: 中间件
  Mfzf : Inport
  Jz : Inport  Port=2
  C1 : Inport  Port=3
  f : Inport  Port=4
  Wz : Inport  Port=5
  Add{,1..2,4} (4 alike) : Sum  Inputs=+-
  Add3 : Sum
  Constant : Constant  Value=0
  Fcn : Fcn  Expr=1/u
  Fcn1 : Fcn  Expr=1+u
  Fcn2 : Fcn  Expr=u^2
  Integrator : Integrator
  Product{,1..2,4..5} (5 alike) : Product
  Product3 : Product  Inputs=3
  Subsystem : Subsystem
  Switch{,1..3} (4 alike) : Switch
  Mr : Outport
  Lr : Outport  Port=2
  C2 : Outport  Port=3
  wires:
  C1/1 -> Switch3/1, Product/2, Add/1
  f/1 -> Subsystem/1(f), Fcn1/1
  Fcn1/1 -> Product1/2
  Product1/1 -> Switch1/1
  Switch1/1 -> Add4/2
  Mfzf/1 -> Add2/1, Add4/1, Switch2/1
  Add2/1 -> Product5/2
  Fcn/1 -> Product5/1
  Switch2/1 -> Mr/1
  Jz/1 -> Product/1, Subsystem/2(Jz), Fcn/1
  Wz/1 -> Fcn2/1, Product4/2
  Fcn2/1 -> Product3/3
  Integrator/1 -> Lr/1, Switch3/2, Switch2/2, Switch1/2, Switch/2
  Product3/1 -> Switch/1
  Constant/1 -> Switch/3
  Add1/1 -> Add3/1
  Switch/1 -> Add3/2
  Add3/1 -> Product1/1, Switch1/3
  Product/1 -> Add1/2
  Product2/1 -> Add1/1
  Add/1 -> Product2/2
  Subsystem/4(Cp) -> Product4/1
  Subsystem/3(Kcp2) -> Product3/2
  Subsystem/1(J) -> Product2/1
  Subsystem/2(Tc) -> Product3/1
  Product4/1 -> Integrator/1
  Add4/1 -> Switch2/3, Add2/2
  Switch3/1 -> Add/2, C2/1
  Product5/1 -> Switch3/3

== system COGAG/sss2/Subsystem2 ==
  note: 从动件
  Mr : Inport
  J2 : Inport  Port=2
  C2 : Inport  Port=3
  n2in : Inport  Port=4
  Add : Sum  Inputs=+-
  Add1 : Sum
  Fcn : Fcn  Expr=30*u/pi
  Integrator : Integrator
  Product : Product
  M2 : Outport
  n2 : Outport  Port=2
  wires:
  Mr/1 -> Add/1
  Add/1 -> M2/1
  J2/1 -> Product/1
  C2/1 -> Fcn/1, Product/2
  Fcn/1 -> Integrator/1
  Integrator/1 -> Add1/1
  n2in/1 -> Add1/2
  Add1/1 -> n2/1
  Product/1 -> Add/2

== system COGAG/sss2/Subsystem3 ==
  note: 主动件
  M1 : Inport
  n1 : Inport  Port=2
  J1 : Inport  Port=3
  Derivative : Derivative
  Fcn2 : Fcn  Expr=u*pi/30
  Product : Product
  Sum : Sum  Inputs=|+-
  Mfzf : Outport
  wf : Outport  Port=2
  C1 : Outport  Port=3
  wires:
  n1/1 -> Fcn2/1
  Fcn2/1 -> wf/1, Derivative/1
  M1/1 -> Sum/1
  J1/1 -> Product/2
  Product/1 -> Sum/2
  Sum/1 -> Mfzf/1
  Derivative/1 -> C1/1, Product/1

== system COGAG/GT1/HC/Subsystem1 ==
  Gin : Inport
  Pin : Inport  Port=2
  Tin : Inport  Port=3
  Divide : Product  Inputs=*/
  Divide1 : Product  Inputs=*/
  Divide2 : Product  Inputs=*/
  Fcn : Fcn  Expr=sqrt(u)
  P0 : Constant  Value=100000
  Product : Product  RndMeth=Zero
  T0 : Constant  Value=288
  Gz : Outport
  wires:
  Tin/1 -> Divide/1
  T0/1 -> Divide/2
  Divide/1 -> Fcn/1
  Pin/1 -> Divide1/1
  P0/1 -> Divide1/2
  Gin/1 -> Divide2/1
  Divide1/1 -> Divide2/2
  Fcn/1 -> Product/1
  Divide2/1 -> Product/2
  Product/1 -> Gz/1

== system COGAG/GT1/HC/Subsystem2 ==
  Gz : Inport
  nz : Inport  Port=2
  Lookup Table (2-D) : Lookup2D  RowIndex=[6000 6300 6500 6800 7000 7300 7500 7800]  ColumnIndex=[12:0.2:29]  Table=|
      | [2.4803 2.5510 2.6217 2.6924 2.7630 2.8337 2.9044 2.9751 3.0172 2.9863 2.9541 2.9206 2.8860 2.8500 2.8129 2.7745 2.7349 2.6940 2.6519 2.6085 2.5640 2.5181 2.4711 2.4906 2.5237 2.5573 2.5913 2.6257 2.6605 2.6958 2.7314 2.7675 2.8040 2.8409 2.8783 2.9161 2.9543 2.9929 3.0319 3.0714 3.1112 3.1515 3.1923 3.2334 3.2750 3.3169 3.3593 3.4022 3.4454 3.4891 3.5332 3.5777 3.6226 3.6679 3.7137 3.7599 3.8065 3.8535 3.9010 3.9488 3.9971 4.0307 4.0450 4.0645  4.0889 4.0613 4.0669 4.0759 4.0882 4.1107 4.1332 4.1561 4.2095 4.2632 4.3174 4.3720 4.4271 4.4825 4.5384 4.5947 4.6514 4.7085 4.7660 4.8240 4.8824 5.0412;
      | 2.4803 2.5510 2.6217 2.6924 2.7630 2.8337 2.9044 2.9751 3.0457 3.1164 3.1871 3.2578 3.3284 3.3991 3.5124 3.4922 3.4694 3.4440 3.4159 3.3853 3.3520 3.3161 3.2775 3.2364 3.1926 3.1462 3.0972 3.0456 2.9914 2.9345 2.8750 2.8129 2.8040 2.8409 2.8783 2.9161 2.9543 2.9929 3.0319 3.0714 3.1112 3.1515 3.1923 3.2334 3.2750 3.3169 3.3593 3.4022 3.4454 3.4891 3.5332 3.5777 3.6226 3.6679 3.7137 3.7599 3.8065 3.8535 3.9010 3.9488 3.9971 4.0307 4.0450 4.0645  4.0889 4.0613 4.0669 4.0759 4.0882 4.1107 4.1332 4.1561 4.2095 4.2632 4.3174 4.3720 4.4271 4.4825 4.5384 4.5947 4.6514 4.7085 4.7660 4.8240 4.8824 5.0412;
      | 2.4803 2.5510 2.6217 2.6924 2.7630 2.8337 2.9044 2.9751 3.0457 3.1164 3.1871 3.2578 3.3284 3.3991 3.4698 3.5405 3.6111 3.6818 3.7525 3.8394 3.8358 3.8266 3.8119 3.7916 3.7659 3.7345 3.6977 3.6553 3.6073 3.5539 3.4948 3.4303 3.3602 3.2845 3.2034 3.1167 3.0244 2.9929 3.0319 3.0714 3.1112 3.1515 3.1923 3.2334 3.2750 3.3169 3.3593 3.4022 3.4454 3.4891 3.5332 3.5777 3.6226 3.6679 3.7137 3.7599 3.8065 3.8535 3.9010 3.9488 3.9971 4.0307 4.0450 4.0645  4.0889 4.0613 4.0669 4.0759 4.0882 4.1107 4.1332 4.1561 4.2095 4.2632 4.3174 4.3720 4.4271 4.4825 4.5384 4.5947 4.6514 4.7085 4.7660 4.8240 4.8824 5.0412;
      | 2.4803 2.5510 2.6217 2.6924 2.7630 2.8337 2.9044 2.9751 3.0457 3.1164 3.1871 3.2578 3.3284 3.3991 3.4698 3.5405 3.6111 3.6818 3.7525 3.8231 3.8938 3.9645 4.0352 4.1058 4.1765 4.2472 4.3179 4.4049 4.4021 4.3892 4.3664 4.3334 4.2904 4.2374 4.1744 4.1012 4.0181 3.9249 3.8216 3.7083 3.5850 3.4516 3.3082 3.2334 3.2750 3.3169 3.3593 3.4022 3.4454 3.4891 3.5332 3.5777 3.6226 3.6679 3.7137 3.7599 3.8065 3.8535 3.9010 3.9488 3.9971 4.0307 4.0450 4.0645  4.0889 4.0613 4.0669 4.0759 4.0882 4.1107 4.1332 4.1561 4.2095 4.2632 4.3174 4.3720 4.4271 4.4825 4.5384 4.5947 4.6514 4.7085 4.7660 4.8240 4.8824 5.0412;
      | 2.4803 2.5510 2.6217 2.6924 2.7630 2.8337 2.9044 2.9751 3.0457 3.1164 3.1871 3.2578 3.3284 3.3991 3.4698 3.5405 3.6111 3.6818 3.7525 3.8231 3.8938 3.9645 4.0352 4.1058 4.1765 4.2472 4.3179 4.3885 4.4592 4.5299 4.6006 4.6379 4.6228 4.5996 4.5680 4.5283 4.4803 4.4241 4.3596 4.2869 4.2060 4.1168 4.0195 3.9138 3.8000 3.6779 3.5476 3.4090 3.4054 3.4591 3.5000 3.5277 3.5426 3.5679 3.5837 3.5999 3.8065 3.8535 3.9010 3.9488 3.9971 4.0307 4.0450 4.0645  4.0889 4.0613 4.0669 4.0759 4.0882 4.1107 4.1332 4.1561 4.2095 4.2632 4.3174 4.3720 4.4271 4.4825 4.5384 4.5947 4.6514 4.7085 4.7660 4.8240 4.8824 5.0412;
      | 2.4803 2.5510 2.6217 2.6924 2.7630 2.8337 2.9044 2.9751 3.0457 3.1164 3.1871 3.2578 3.3284 3.3991 3.4698 3.5405 3.6111 3.6818 3.7525 3.8231 3.8938 3.9645 4.0352 4.1058 4.1765 4.2472 4.3179 4.3885 4.4592 4.5299 4.6006 4.6712 4.7419 4.8126 4.8833 4.9539 5.0246 5.0953 5.1660 5.2000 5.1000 5.0000 4.9700 4.9000 4.8200 4.6810 4.6468 4.6015 4.5451 4.4775 4.3988 4.3090 4.2081 4.0961 3.9729 3.8386 3.8065 3.8535 3.9010 3.9488 3.9971 4.0307 4.0450 4.0645  4.0889 4.0613 4.0669 4.0759 4.0882 4.1107 4.1332 4.1561 4.2095 4.2632 4.3174 4.3720 4.4271 4.4825 4.5384 4.5947 4.6514 4.7085 4.7660 4.8240 4.8824 5.0412;
      | 2.4803 2.5510 2.6217 2.6924 2.7630 2.8337 2.9044 2.9751 3.0457 3.1164 3.1871 3.2578 3.3284 3.3991 3.4698 3.5405 3.6111 3.6818 3.7525 3.8231 3.8938 3.9645 4.0352 4.1058 4.1765 4.2472 4.3179 4.3885 4.4592 4.5299 4.6006 4.6712 4.7419 4.8126 4.8833 4.9539 5.0246 5.0953 5.1660 5.2366 5.3073 5.3780 5.4486 5.5193 5.5000 5.4500 5.4000 5.3500 5.3000 5.2500 5.2036 5.1763 5.1322 5.0715 4.9940 4.8998 4.7889 4.6613 4.5169 4.3559 4.0182 4.0307 4.0450 4.0645 4.0889 4.0613 4.0669 4.0759 4.0882 4.1107 4.1332 4.1561 4.2095 4.2632 4.3174 4.3720 4.4271 4.4825 4.5384 4.5947 4.6514 4.7085 4.7660 4.8240 4.8824 5.0412; 
      | 2.4803 2.5510 2.6217 2.6924 2.7630 2.8337 2.9044 2.9751 3.0457 3.1164 3.1871 3.2578 3.3284 3.3991 3.4698 3.5405 3.6111 3.6818 3.7525 3.8231 3.8938 3.9645 4.0352 4.1058 4.1765 4.2472 4.3179 4.3885 4.4592 4.5299 4.6006 4.6712 4.7419 4.8126 4.8833 4.9539 5.0246 5.0953 5.1660 5.2366 5.3073 5.3780 5.4486 5.5193 5.5900 5.6607 5.7313 5.8020 5.8727 5.9434 6.0140 6.0847 6.1554 6.2261 6.2967 6.3674 6.4381 6.5088 5.5861 5.3841 5.1514 4.8878 4.5936 4.0685 4.0889 4.0613 4.0669 4.0759 4.0882 4.1107 4.1332 4.1561 4.2095 4.2632 4.3174 4.3720 4.4271 4.4825 4.5384 4.5947 4.6514 4.7085 4.7660 4.8240 4.8824 5.0412;]
  Lookup Table (2-D)1 : Lookup2D  RowIndex=[6000 6300 6500 6800 7000 7300 7500 7800]  ColumnIndex=[12:0.2:29]  Table=|
      | [0.8450 0.8455 0.8460 0.8465 0.8470 0.8480 0.8490 0.8495 0.8500 0.8510 0.8520 0.8530 0.8540 0.8540 0.8540 0.8525 0.8510 0.8500 0.8490 0.8480 0.8470 0.8460 0.8450 0.8455 0.8460 0.8460 0.8460 0.8470 0.8480 0.8480 0.8480 0.8480 0.8480 0.8485 0.8490 0.8490 0.8490 0.8490 0.8490 0.8490 0.8490 0.8490 0.8490 0.8490 0.8490 0.8490 0.8490 0.8490 0.8490 0.8495 0.8500 0.8500 0.8500 0.8500 0.8500 0.8500 0.8500 0.8495 0.8490 0.8495 0.8500 0.8490 0.8480 0.8480 0.8480 0.8475 0.8470 0.8465 0.8460 0.8455 0.8450 0.8445 0.8440 0.8435 0.8430 0.8425 0.8420 0.8415 0.8410 0.8405 0.8400 0.8395 0.8390 0.8385 0.8380 0.8375;
      | 0.8450 0.8455 0.8460 0.8465 0.8470 0.8480 0.8490 0.8495 0.8500 0.8505 0.8510 0.8515 0.8520 0.8520 0.8520 0.8556 0.8597 0.8631 0.8658 0.8678 0.8691 0.8697 0.8696 0.8688 0.8672 0.8650 0.8621 0.8585 0.8542 0.8492 0.8435 0.8371 0.8480 0.8485 0.8490 0.8490 0.8490 0.8490 0.8490 0.8490 0.8490 0.8490 0.8490 0.8490 0.8490 0.8490 0.8490 0.8490 0.8490 0.8495 0.8500 0.8500 0.8500 0.8500 0.8500 0.8500 0.8500 0.8495 0.8490 0.8495 0.8500 0.8490 0.8480 0.8480 0.8480 0.8475 0.8470 0.8465 0.8460 0.8455 0.8450 0.8445 0.8440 0.8435 0.8430 0.8425 0.8420 0.8415 0.8410 0.8405 0.8400 0.8395 0.8390 0.8385 0.8380 0.8375;
      | 0.8450 0.8455 0.8460 0.8465 0.8470 0.8480 0.8490 0.8495 0.8500 0.8505 0.8510 0.8515 0.8520 0.8520 0.8520 0.8525 0.8530 0.8530 0.8530 0.8611 0.8688 0.8754 0.8809 0.8854 0.8888 0.8910 0.8922 0.8923 0.8914 0.8893 0.8861 0.8819 0.8766 0.8702 0.8627 0.8541 0.8444 0.8490 0.8490 0.8490 0.8490 0.8490 0.8490 0.8490 0.8490 0.8490 0.8490 0.8490 0.8490 0.8495 0.8500 0.8500 0.8500 0.8500 0.8500 0.8500 0.8500 0.8495 0.8490 0.8495 0.8500 0.8490 0.8480 0.8480 0.8480 0.8475 0.8470 0.8465 0.8460 0.8455 0.8450 0.8445 0.8440 0.8435 0.8430 0.8425 0.8420 0.8415 0.8410 0.8405 0.8400 0.8395 0.8390 0.8385 0.8380 0.8375;
      | 0.8450 0.8455 0.8460 0.8465 0.8470 0.8480 0.8490 0.8495 0.8500 0.8505 0.8510 0.8515 0.8520 0.8520 0.8520 0.8525 0.8530 0.8530 0.8530 0.8540 0.8550 0.8565 0.8580 0.8600 0.8620 0.8630 0.8640 0.8669 0.8710 0.8830 0.8930 0.9010 0.9070 0.9110 0.9129 0.9129 0.9108 0.9067 0.9006 0.8925 0.8824 0.8703 0.8561 0.8490 0.8490 0.8490 0.8490 0.8490 0.8490 0.8495 0.8500 0.8500 0.8500 0.8500 0.8500 0.8500 0.8500 0.8495 0.8490 0.8495 0.8500 0.8490 0.8480 0.8480 0.8480 0.8475 0.8470 0.8465 0.8460 0.8455 0.8450 0.8445 0.8440 0.8435 0.8430 0.8425 0.8420 0.8415 0.8410 0.8405 0.8400 0.8395 0.8390 0.8385 0.8380 0.8375;
      | 0.8450 0.8455 0.8460 0.8465 0.8470 0.8480 0.8490 0.8495 0.8500 0.8505 0.8510 0.8515 0.8520 0.8520 0.8520 0.8525 0.8530 0.8530 0.8530 0.8540 0.8550 0.8565 0.8580 0.8600 0.8620 0.8630 0.8640 0.8505 0.8500 0.8500 0.8500 0.8499 0.8618 0.8720 0.8808 0.8879 0.8935 0.8975 0.8999 0.9008 0.9001 0.8978 0.8940 0.8886 0.8816 0.8731 0.8630 0.8513 0.8490 0.8495 0.8500 0.8500 0.8500 0.8500 0.8500 0.8500 0.8500 0.8495 0.8490 0.8495 0.8500 0.8490 0.8480 0.8480 0.8480 0.8475 0.8470 0.8465 0.8460 0.8455 0.8450 0.8445 0.8440 0.8435 0.8430 0.8425 0.8420 0.8415 0.8410 0.8405 0.8400 0.8395 0.8390 0.8385 0.8380 0.8375;
      | 0.8450 0.8455 0.8460 0.8465 0.8470 0.8480 0.8490 0.8495 0.8500 0.8505 0.8510 0.8515 0.8520 0.8520 0.8520 0.8525 0.8530 0.8530 0.8530 0.8540 0.8550 0.8565 0.8580 0.8600 0.8620 0.8630 0.8640 0.8505 0.8500 0.8500 0.8500 0.8495 0.8490 0.8485 0.8480 0.8475 0.8470 0.8470 0.8470 0.8586 0.8661 0.8726 0.8781 0.8825 0.8860 0.8884 0.8897 0.8901 0.8894 0.8878 0.8851 0.8813 0.8766 0.8708 0.8640 0.8562 0.8500 0.8495 0.8490 0.8495 0.8500 0.8490 0.8480 0.8480 0.8480 0.8475 0.8470 0.8465 0.8460 0.8455 0.8450 0.8445 0.8440 0.8435 0.8430 0.8425 0.8420 0.8415 0.8410 0.8405 0.8400 0.8395 0.8390 0.8385 0.8380 0.8375;
      | 0.8450 0.8455 0.8460 0.8465 0.8470 0.8480 0.8490 0.8495 0.8500 0.8505 0.8510 0.8515 0.8520 0.8520 0.8520 0.8525 0.8530 0.8530 0.8530 0.8540 0.8550 0.8565 0.8580 0.8600 0.8620 0.8630 0.8640 0.8505 0.8500 0.8500 0.8500 0.8495 0.8490 0.8485 0.8480 0.8475 0.8470 0.8470 0.8470 0.8465 0.8460 0.8455 0.8450 0.8450 0.8450 0.8460 0.8456 0.8496 0.8528 0.8554 0.8572 0.8582 0.8585 0.8581 0.8569 0.8550 0.8523 0.8500 0.8500 0.8495 0.8495 0.8490 0.8480 0.8480 0.8480 0.8475 0.8470 0.8465 0.8460 0.8455 0.8450 0.8445 0.8440 0.8435 0.8430 0.8425 0.8420 0.8415 0.8410 0.8405 0.8400 0.8395 0.8390 0.8385 0.8380 0.8375;
      | 0.8450 0.8455 0.8460 0.8465 0.8470 0.8480 0.8490 0.8495 0.8500 0.8505 0.8510 0.8515 0.8520 0.8520 0.8520 0.8525 0.8530 0.8530 0.8530 0.8540 0.8550 0.8565 0.8580 0.8600 0.8620 0.8630 0.8640 0.8505 0.8500 0.8500 0.8500 0.8495 0.8490 0.8485 0.8480 0.8475 0.8470 0.8470 0.8470 0.8465 0.8460 0.8455 0.8450 0.8450 0.8450 0.8445 0.8440 0.8445 0.8450 0.8445 0.8440 0.8425 0.8400 0.8415 0.8430 0.8455 0.8480 0.8510 0.8550 0.8600 0.8650 0.8650 0.8650 0.8650 0.8480 0.8475 0.8470 0.8465 0.8460 0.8455 0.8450 0.8445 0.8440 0.8435 0.8430 0.8425 0.8420 0.8415 0.8410 0.8405 0.8400 0.8395 0.8390 0.8385 0.8380 0.8375;]
  pi : Outport
  eta : Outport  Port=2
  wires:
  nz/1 -> Lookup Table (2-D)/1, Lookup Table (2-D)1/1
  Gz/1 -> Lookup Table (2-D)1/2, Lookup Table (2-D)/2
  Lookup Table (2-D)/1 -> pi/1
  Lookup Table (2-D)1/1 -> eta/1

== system COGAG/GT1/HC/compresser_TN ==
  Gin : Inport
  Pi : Inport  Port=2
  eta : Inport  Port=3
  Tin : Inport  Port=4
  Add : Sum  Inputs=+-
  Add1 : Sum
  Constant : Constant
  Divide : Product  Inputs=/*
  Fcn : Fcn  Expr=u[1]^(u[2])
  K : Subsystem
  K1 : Constant  Value=1.35
  Mux : Mux  Inputs=2
  Product : Product  Inputs=4  RndMeth=Zero
  Product1 : Product  RndMeth=Zero
  Scope3 : Scope
      settings: YMin=2829.54  YMax=3127.38  SaveName=ScopeData18
  m : Fcn  Expr=(u-1)/u
  Tout : Outport
  Nout : Outport  Port=2
  wires:
  Tin/1 -> K/1(T1), Product1/2, Product/4
  Pi/1 -> Mux/1
  m/1 -> Mux/2
  Mux/1 -> Fcn/1
  Fcn/1 -> Add/1
  Add/1 -> Divide/2
  Divide/1 -> Add1/1, Product/1
  Constant/1 -> Add/2, Add1/2
  Product1/1 -> Tout/1, Scope3/1
  Product/1 -> Nout/1
  Add1/1 -> Product1/1
  K/2(Cp) -> Product/2
  Gin/1 -> Product/3
  eta/1 -> Divide/1
  K1/1 -> m/1

== system COGAG/GT1/HC/zhehe ==
  n : Inport
  Tin : Inport  Port=2
  Divide : Product  Inputs=*/
  Fcn : Fcn  Expr=sqrt(u/288)
  nz : Outport
  wires:
  Tin/1 -> Fcn/1
  n/1 -> Divide/1
  Fcn/1 -> Divide/2
  Divide/1 -> nz/1

== system COGAG/GT1/HT/turbine_TN ==
  Pi : Inport
  eta : Inport  Port=2
  Tin : Inport  Port=3
  Gin : Inport  Port=4
  Add : Sum  Inputs=-+
  Add1 : Sum  Inputs=-+
  Constant : Constant
  Fcn : Fcn  Expr=1/(u[1]^u[2])
  K : Subsystem
  K1 : Constant  Value=1.33
  Mux : Mux  Inputs=2
  Product : Product  Inputs=4  RndMeth=Zero
  Product1 : Product  RndMeth=Zero
  Product2 : Product  RndMeth=Zero
  m : Fcn  Expr=(u-1)/u
  Tout : Outport
  Nout : Outport  Port=2
  wires:
  Tin/1 -> K/1(T1), Product1/2, Product/4
  Pi/1 -> Mux/1
  m/1 -> Mux/2
  Mux/1 -> Fcn/1
  Fcn/1 -> Add/1
  Add/1 -> Product2/2
  eta/1 -> Product2/1
  Product2/1 -> Add1/1, Product/1
  Constant/1 -> Add/2, Add1/2
  Product1/1 -> Tout/1
  Product/1 -> Nout/1
  Add1/1 -> Product1/1
  K/2(Cp) -> Product/2
  Gin/1 -> Product/3
  K1/1 -> m/1

== system COGAG/GT1/LC/Subsystem1 ==
  Gin : Inport
  Pin : Inport  Port=2
  Tin : Inport  Port=3
  Divide : Product  Inputs=*/
  Divide1 : Product  Inputs=*/
  Divide2 : Product  Inputs=*/
  Fcn : Fcn  Expr=sqrt(u)
  P0 : Constant  Value=100000
  Product : Product  RndMeth=Zero
  T0 : Constant  Value=288
  Gz : Outport
  wires:
  Tin/1 -> Divide/1
  T0/1 -> Divide/2
  Divide/1 -> Fcn/1
  Pin/1 -> Divide1/1
  P0/1 -> Divide1/2
  Gin/1 -> Divide2/1
  Divide1/1 -> Divide2/2
  Fcn/1 -> Product/1
  Divide2/1 -> Product/2
  Product/1 -> Gz/1
